simulink model "sl_ibvs"  (R2016b)
settings: Solver=ode45  StartTime=0.0  StopTime=10  RelTol=1e-3  EnableMultiTasking=on
InitFcn:
  | camera = CentralCamera('default')
undefined symbols (not defined in the file or in its folder): mkgrid, transl, trotz
libraries: roblocks x6
settings Model: ExtModeTrigMode=oneshot  ExtModeArmWhenConnect=off  Creator=pic  LastModifiedBy=corkep
settings DataIOCC: SaveFormat=Structure  SignalLoggingSaveFormat=ModelDataLogs  ReturnWorkspaceOutputs=on
settings OptimizationCC: BlockReduction=off  BooleanDataType=off  ExpressionDepthLimit=2147483647  InitFltsAndDblsToZero=on  LifeSpan=inf
settings DebuggingCC: SaveWithParameterizedLinksMsg=none  UnderspecifiedInitializationDetection=Classic  MergeDetectMultiDrivingBlocksExec=none  SignalResolutionControl=TryResolveAllWithWarning  MultiTaskDSMMsg=warning  MultiTaskCondExecSysMsg=none  FcnCallInpInsideContextMsg=warning  AllowSymbolicDim=off  StateNameClashWarn=warning  SFUnexpectedBacktrackingDiag=warning  SFNoUnconditionalDefaultTransitionDiag=warning  SFExecutionAtInitializationDiag=none
settings HardwareCC: ProdBitPerPointer=32  ProdBitPerSizeT=32  ProdBitPerPtrDiffT=32  ProdLargestAtomicFloat=None  ProdIntDivRoundTo=Undefined  ProdEndianess=Unspecified  ProdWordSize=32  ProdHWDeviceType=32-bit Generic  TargetUnknown=on
settings ModelReferenceCC: PropagateSignalLabelsOutOfModel=off
settings GRTTargetCC: TargetLangStandard=C89/C90 (ANSI)  ModelReferenceCompliant=off  CompOptLevelCompliant=off  GeneratePreprocessorConditionals=Disable all  CombineOutputUpdateFcns=off  MatFileLogging=off  GRTInterface=on
settings ConfigComp: CovMetricSettings=dw  CovHtmlReporting=on  CovSaveCumulativeToWorkspaceVar=on  CovSaveSingleToWorkspaceVar=on  CovExternalEMLEnable=off

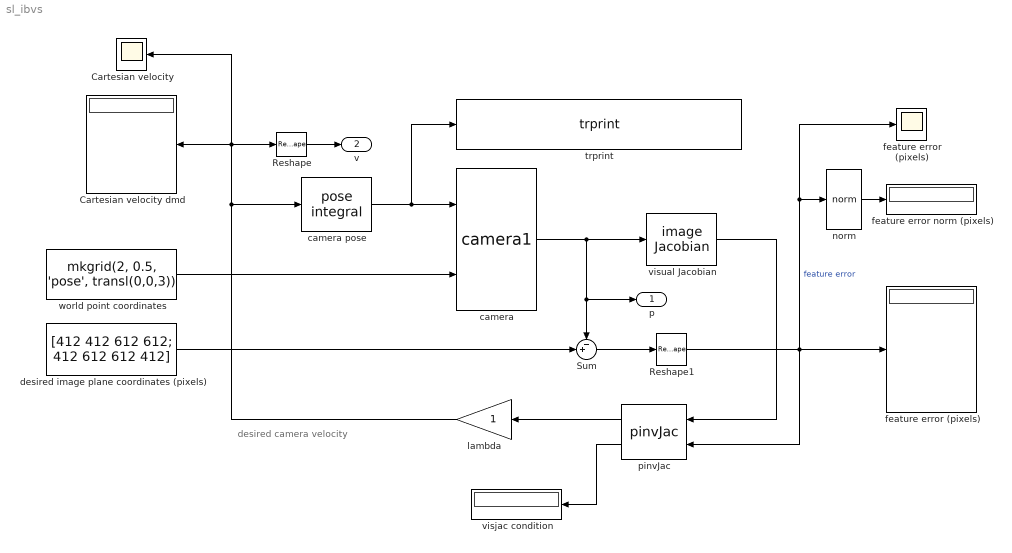
== system sl_ibvs ==
  note: desired camera velocity
  Cartesian velocity : Scope
  Cartesian velocity dmd : Display
      settings: Format=bank
  Reshape : Reshape  OutputDimensions=6
  Reshape1 : Reshape  OutputDimensions=6
  Sum : Sum  Inputs=-+|  SaturateOnIntegerOverflow=on  InputSameDT=on  OutDataTypeStr=Inherit: Same as first input
  camera : roblocks/Vision/camera1  cam=camera
  camera pose : roblocks/Toolbox/pose integral  T0=transl(0,0,1)*trotz(1.5)  dt=0.02
  desired image plane coordinates (pixels) : Constant  Value=[412 412 612 612; 412 612 612 412]  VectorParams1D=off
  feature error norm (pixels) : Display
  feature error (pixels) : Display
      settings: Format=bank
  "feature error (pixels) " : Scope
  lambda : Gain  SaturateOnIntegerOverflow=on  OutDataTypeStr=Inherit: Same as input  ParamDataTypeStr=Inherit: Same as input
  norm : roblocks/Toolbox/norm  SystemSampleTime=-1
  pinvJac : roblocks/Toolbox/pinvJac
  trprint : roblocks/Toolbox/trprint  options={}
      link override S-Function: Parameters=options
  visjac condition : Display
  visual Jacobian : roblocks/Vision/image Jacobian  cam=camera  z=3
  world point coordinates : Constant  Value=mkgrid(2, 0.5, 'pose', transl(0,0,3))  VectorParams1D=off
  p : Outport
  v : Outport  Port=2
  wires:
  Sum/1 -> Reshape1/1
  desired image plane coordinates (pixels)/1 -> Sum/2
  Reshape1/1 -> feature error (pixels)/1, pinvJac/2, "feature error (pixels) "/1, norm/1  "feature error"
  pinvJac/2 -> visjac condition/1
  pinvJac/1 -> lambda/1
  camera pose/1 -> trprint/1, camera/1
  visual Jacobian/1 -> pinvJac/1
  lambda/1 -> Cartesian velocity/1, Reshape/1, Cartesian velocity dmd/1, camera pose/1
  Reshape/1 -> v/1
  camera/1 -> visual Jacobian/1, Sum/1, p/1
  world point coordinates/1 -> camera/2
  norm/1 -> feature error norm (pixels)/1
